simulink model "blank_canvas_135_SLRT"  (R2025b)
settings: Solver=FixedStepDiscrete  StartTime=0.0  StopTime=2  FixedStep=Ts  RelTol=1e-3
libraries: slrealtimeloglib x1, slrealtimetgmanagement x1
settings Model: Creator=gdudgeon  LastModifiedBy=gdudgeon
settings SolverCC: ConcurrentTasks=on  PositivePriorityOrder=on
settings DataIOCC: SaveOutput=off  SignalLogging=off  DSMLogging=off  SaveTime=off  ReturnWorkspaceOutputs=off
settings OptimizationCC: BlockReduction=off  OptimizeBlockIOStorage=off
settings DebuggingCC: TasksWithSamePriorityMsg=none
settings HardwareCC: ProdBitPerLong=64.0  ProdLongLongMode=on  ProdHWDeviceType=Intel->x86-64 (Linux 64)
settings RTWCC: SystemTargetFile=speedgoat.tlc  TemplateMakefile=slrealtime_default_tmf  Toolchain=Simulink Real-Time Toolchain  BuildConfiguration=Faster Runs  CodeExecutionProfiling=on  TargetLang=C++  GPUComputeCapability=3.5  Description=Speedgoat Real-Time Target Machine
settings SimulinkRealTimeTargetCC: SLRTFileLogMaxRuns=1.0  ExtModeMaxTrigDuration=10.0  ExtModeStaticAllocSize=1000000.0  ExtModeTransport=0.0  MultiwordLength=2048.0  DynamicStringBufferSize=256.0  PreserveMATLABNamespacesInGeneratedCode=on  SubcomponentCodeInterfacePackaging=Reusable function  MATLABClassNameForMDSCustomization=Simulink.SoftwareTarget.GRTCustomization  InstructionSetFMA=off  LogToMDFFile=off

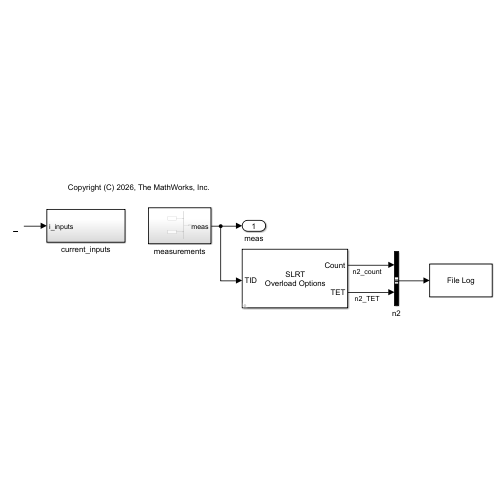
[thumbnail: Simulink's stored preview of the top-level diagram]
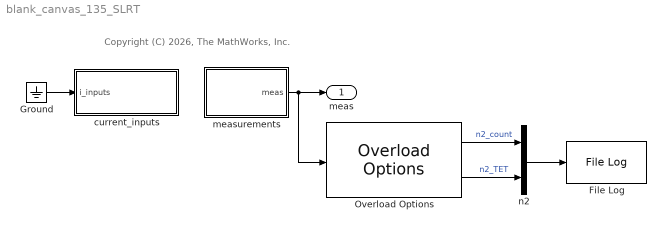
== system blank_canvas_135_SLRT ==
  note: Copyright (C) 2026, The MathWorks, Inc.
  File Log : slrealtimeloglib/File Log  decimation=1  inputProcessing=Elements as channels (sample based)
  Ground : Ground
  Overload Options : slrealtimetgmanagement/Overload Options  startupDur=5  startupDurSrc=Tunable Parameter  maxOverload=1000  maxOverloadSrc=Tunable Parameter  TETFlag=on
  current_inputs : Subsystem
  measurements : Subsystem
  n2 : BusCreator  Inputs=2
  meas : Outport
  wires:
  measurements/1(meas) -> Overload Options/1, meas/1
  Ground/1 -> current_inputs/1(i_inputs)
  Overload Options/1 -> n2/1  "n2_count"
  Overload Options/2 -> n2/2  "n2_TET"
  n2/1 -> File Log/1

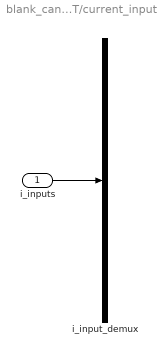
== system blank_canvas_135_SLRT/current_inputs ==
  i_inputs : Inport
  i_input_demux : Demux  Outputs=2
  wires:
  i_inputs/1 -> i_input_demux/1

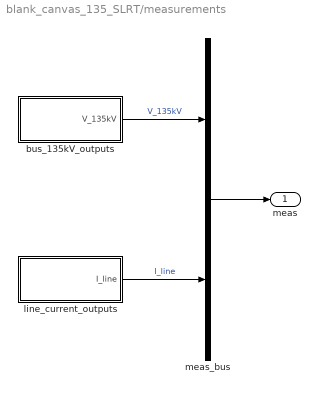
== system blank_canvas_135_SLRT/measurements ==
  bus_135kV_outputs : Subsystem
  line_current_outputs : Subsystem
  meas_bus : BusCreator  Inputs=2
  meas : Outport
  wires:
  meas_bus/1 -> meas/1
  line_current_outputs/1(I_line) -> meas_bus/2  "I_line"
  bus_135kV_outputs/1(V_135kV) -> meas_bus/1  "V_135kV"

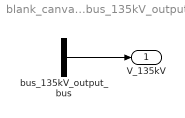
== system blank_canvas_135_SLRT/measurements/bus_135kV_outputs ==
  bus_135kV_output_bus : BusCreator  Inputs=2
  V_135kV : Outport  VectorParamsAs1DForOutWhenUnconnected=off
  wires:
  bus_135kV_output_bus/1 -> V_135kV/1

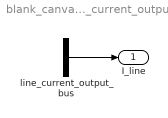
== system blank_canvas_135_SLRT/measurements/line_current_outputs ==
  line_current_output_bus : BusCreator  Inputs=2
  I_line : Outport  VectorParamsAs1DForOutWhenUnconnected=off
  wires:
  line_current_output_bus/1 -> I_line/1
